simulink model "PID_ZieglerNichols"  (R2024a)
settings: Solver=ode3  StartTime=0.0  StopTime=100  FixedStep=0.1  RelTol=1e-3  EnableMultiTasking=on
values from neighbouring files (symbols this model uses):
  K_crit = 10.65    [ziegler_nichols_para.m]
  T_crit = 13    [ziegler_nichols_para.m]
settings Model: Creator=gregor  LastModifiedBy=tunkarlu
settings SolverCC: AlgebraicLoopSolver=TrustRegion
settings DataIOCC: LimitDataPoints=on  SaveFormat=Array  SignalLoggingSaveFormat=ModelDataLogs  SaveState=on  ReturnWorkspaceOutputs=off
settings OptimizationCC: ExpressionDepthLimit=2147483647  InitFltsAndDblsToZero=on  LifeSpan=inf
settings DebuggingCC: SaveWithParameterizedLinksMsg=none  UnderspecifiedInitializationDetection=Classic  MergeDetectMultiDrivingBlocksExec=none  SignalResolutionControl=TryResolveAllWithWarning  SolverPrmCheckMsg=warning  MultiTaskDSMMsg=warning  MultiTaskCondExecSysMsg=none  FcnCallInpInsideContextMsg=warning  UnconnectedInputMsg=warning  UnconnectedOutputMsg=warning  UnconnectedLineMsg=warning  StateNameClashWarn=warning  SFUnexpectedBacktrackingDiag=warning  SFNoUnconditionalDefaultTransitionDiag=warning  ArithmeticOperatorsInVariantConditions=warning
settings HardwareCC: ProdBitPerPointer=32  ProdBitPerSizeT=32  ProdBitPerPtrDiffT=32  ProdLargestAtomicFloat=None  ProdIntDivRoundTo=Undefined  ProdEndianess=Unspecified  ProdWordSize=32  ProdHWDeviceType=32-bit Generic
settings ModelReferenceCC: EnableRefExpFcnMdlSchedulingChecks=on  PropagateSignalLabelsOutOfModel=off
settings SFSimCC: SimUseLocalCustomCode=off  CustomCodeUndefinedFunction=UseInterfaceOnly
settings RTWCC: RTWUseLocalCustomCode=off  GPUComputeCapability=3.5  DLArmComputeVersion=19.05
settings CodeAppCC: StateflowObjectComments=on
settings GRTTargetCC: TargetFcnLib=ansi_tfl_tmw.mat  TargetLangStandard=C89/C90 (ANSI)  CombineOutputUpdateFcns=off  GRTInterface=on
settings ConfigComp: CovMetricSettings=dw  CovSaveCumulativeToWorkspaceVar=on  CovSaveSingleToWorkspaceVar=on  CovExternalEMLEnable=off

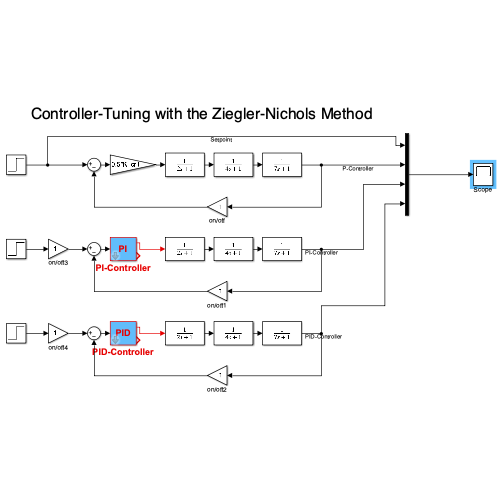
[thumbnail: Simulink's stored preview of the top-level diagram]
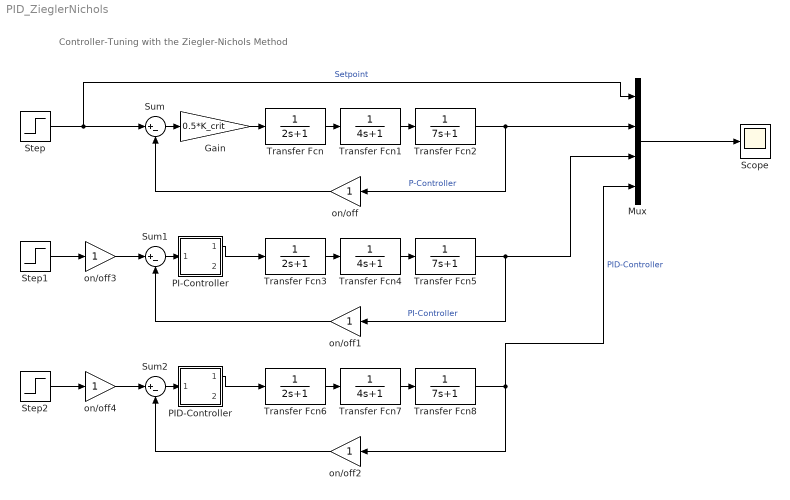
== system PID_ZieglerNichols ==
  note: Controller-Tuning with the Ziegler-Nichols Method
  Gain : Gain  Gain=0.5*K_crit
  Mux : Mux
  PI-Controller : Subsystem  mask{P=0.45*K_crit, I=0.85*T_crit}
      mask prompts: P "Gain (K)"; I "Integral Time (Ti)"
      mask help:
      | PI-Controller:
      |
      | G_C(s) = K(1 + 1/(s*Ti))
      mask Help:
      | PI-Controller:
      | 
      | G_C(s) = K(1 + 1/(s*Ti))
      mask Display: disp('PI');
  PID-Controller : Subsystem  mask{P=0.6*K_crit, I=0.5*T_crit, D=0.12*T_crit}
      mask prompts: P "Gain (K)"; I "Integral Time (Ti)"; D "Derivative Time (Td)"
      mask help:
      | PID-Controller:
      |
      | G_C(s) = K(1 + 1/(s*Ti) + Td*s)
      mask Help:
      | PID-Controller:
      | 
      | G_C(s) = K(1 + 1/(s*Ti) + Td*s)
      mask Display: disp('PID');
  "Scope " : Scope
  Step : Step  SampleTime=0
  Step1 : Step  SampleTime=0
  Step2 : Step  SampleTime=0
  Sum : Sum  Inputs=|+-
  Sum1 : Sum  Inputs=|+-
  Sum2 : Sum  Inputs=|+-
  Transfer Fcn : TransferFcn  Numerator=1  Denominator=[2 1]
  Transfer Fcn1 : TransferFcn  Denominator=[4 1]
  Transfer Fcn2 : TransferFcn  Denominator=[7 1]
  Transfer Fcn3 : TransferFcn  Numerator=1  Denominator=[2 1]
  Transfer Fcn4 : TransferFcn  Denominator=[4 1]
  Transfer Fcn5 : TransferFcn  Denominator=[7 1]
  Transfer Fcn6 : TransferFcn  Numerator=1  Denominator=[2 1]
  Transfer Fcn7 : TransferFcn  Denominator=[4 1]
  Transfer Fcn8 : TransferFcn  Denominator=[7 1]
  on/off{,1..4} (5 alike) : Gain
  wires:
  Transfer Fcn/1 -> Transfer Fcn1/1
  Transfer Fcn1/1 -> Transfer Fcn2/1
  Mux/1 -> "Scope "/1
  Sum/1 -> Gain/1
  Transfer Fcn2/1 -> on/off/1, Mux/2  "P-Controller"
  on/off/1 -> Sum/2
  Transfer Fcn3/1 -> Transfer Fcn4/1
  Transfer Fcn4/1 -> Transfer Fcn5/1
  Sum1/1 -> PI-Controller/1(In_1)
  Transfer Fcn5/1 -> Mux/3, on/off1/1  "PI-Controller"
  PI-Controller/1(Out_1) -> Transfer Fcn3/1
  on/off1/1 -> Sum1/2
  Transfer Fcn6/1 -> Transfer Fcn7/1
  Transfer Fcn7/1 -> Transfer Fcn8/1
  Sum2/1 -> PID-Controller/1(In_1)
  Transfer Fcn8/1 -> Mux/4, on/off2/1  "PID-Controller"
  PID-Controller/1(Out_1) -> Transfer Fcn6/1
  on/off2/1 -> Sum2/2
  Gain/1 -> Transfer Fcn/1
  Step/1 -> Mux/1, Sum/1  "Setpoint"
  Step1/1 -> on/off3/1
  on/off3/1 -> Sum1/1
  Step2/1 -> on/off4/1
  on/off4/1 -> Sum2/1

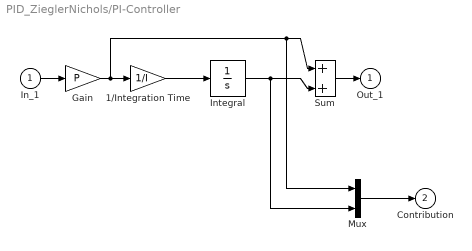
== system PID_ZieglerNichols/PI-Controller ==
  In_1 : Inport
  1/Integration Time : Gain  Gain=1/I  SaturateOnIntegerOverflow=on  OutDataTypeStr=Inherit: Same as input  ParamDataTypeStr=Inherit: Same as input
  Gain : Gain  Gain=P  SaturateOnIntegerOverflow=on  OutDataTypeStr=Inherit: Same as input  ParamDataTypeStr=Inherit: Same as input
  Integral : TransferFcn  Denominator=[1 0]
  Mux : Mux  Inputs=2
  Sum : Sum  InputSameDT=on  SaturateOnIntegerOverflow=on  OutDataTypeStr=Inherit: Same as first input
  Out_1 : Outport  InitialOutput=0
  Contribution : Outport  Port=2  InitialOutput=0
  wires:
  Integral/1 -> Sum/2, Mux/2
  Sum/1 -> Out_1/1
  In_1/1 -> Gain/1
  Gain/1 -> 1/Integration Time/1, Mux/1, Sum/1
  1/Integration Time/1 -> Integral/1
  Mux/1 -> Contribution/1

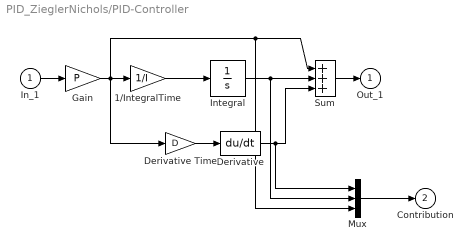
== system PID_ZieglerNichols/PID-Controller ==
  In_1 : Inport
  1/IntegralTime : Gain  Gain=1/I  SaturateOnIntegerOverflow=on  OutDataTypeStr=Inherit: Same as input  ParamDataTypeStr=Inherit: Same as input
  Derivative : Derivative
  Derivative Time : Gain  Gain=D  SaturateOnIntegerOverflow=on  OutDataTypeStr=Inherit: Same as input  ParamDataTypeStr=Inherit: Same as input
  Gain : Gain  Gain=P  SaturateOnIntegerOverflow=on  OutDataTypeStr=Inherit: Same as input  ParamDataTypeStr=Inherit: Same as input
  Integral : TransferFcn  Denominator=[1 0]
  Mux : Mux  Inputs=3
  Sum : Sum  Inputs=+++  InputSameDT=on  SaturateOnIntegerOverflow=on  OutDataTypeStr=Inherit: Same as first input
  Out_1 : Outport  InitialOutput=0
  Contribution : Outport  Port=2  InitialOutput=0
  wires:
  Integral/1 -> Sum/2, Mux/2
  Derivative/1 -> Sum/3, Mux/1
  Sum/1 -> Out_1/1
  Derivative Time/1 -> Derivative/1
  In_1/1 -> Gain/1
  Gain/1 -> 1/IntegralTime/1, Derivative Time/1, Sum/1, Mux/3
  1/IntegralTime/1 -> Integral/1
  Mux/1 -> Contribution/1
